simulink model "schemablocpendule1"  (R2021b)
settings: Solver=VariableStepAuto  StartTime=0.0  StopTime=10.0  RelTol=1e-3
undefined symbols (not defined in the file): a, DiscIntNeverNeededParam, Ki, Ku, Ti
libraries: simulink x5, slctrlblks x1
settings Model: Creator=spaet  LastModifiedBy=eloua

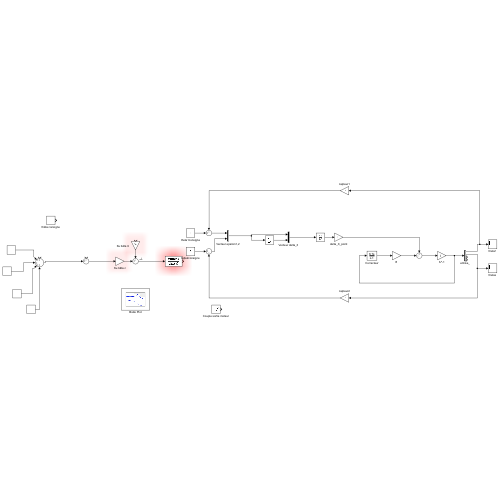
[thumbnail: Simulink's stored preview of the top-level diagram]
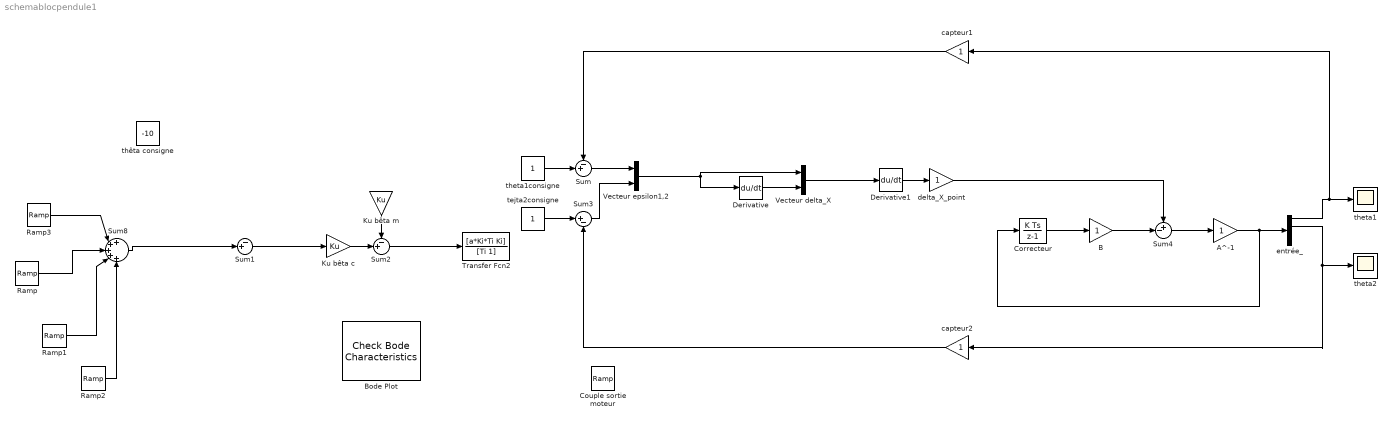
== system schemablocpendule1 ==
  A^-1 : Gain
  B : Gain
  Bode Plot : slctrlblks/Model Verification/Check Bode  Characteristics  InstantiateOnLoad=on  SaveOperatingPoints=off  LinearizationIOs={'/Sum2', 1, 'in', 'on', '';'/TMD sur la caméra', 1, 'out', 'on', ''}  LinearizeAt=SnapshotTimes  SnapshotTimes=[0]  TriggerType=rising  SampleTime=auto  RateConversionMethod=zoh  PreWarpFreq=10  UseExactDelayModel=off  UseFullBlockNameLabels=off  UseBusSignalLabels=off  enabled=on  stopWhenAssertionFail=off  export=off  ViewDlgPos=[137 244 510 390]  OpenViewOnLoad=off  LaunchViewOnOpen=off  FrequencyUnits=rad/s  MagnitudeUnits=dB  PhaseUnits=deg  TimeUnits=seconds  EnableUpperBound=off  UpperBoundFrequencies=[]  UpperBoundMagnitudes=[]  EnableLowerBound=off  LowerBoundFrequencies=[]  LowerBoundMagnitudes=[]
  Correcteur : DiscreteIntegrator  SampleTime=-1  ICPrevOutput=DiscIntNeverNeededParam  ICPrevScaledInput=DiscIntNeverNeededParam
  Couple sortie moteur : simulink/Sources/Ramp  slope=1  start=0  InitialOutput=0
  Derivative : Derivative
  Derivative1 : Derivative
  Ku bêta c : Gain  Gain=Ku
  Ku bêta m : Gain  Gain=Ku
  Ramp : simulink/Sources/Ramp  slope=1  start=0  InitialOutput=0
  Ramp1 : simulink/Sources/Ramp  slope=-1  start=10  InitialOutput=0
  Ramp2 : simulink/Sources/Ramp  slope=-1  start=20  InitialOutput=0
  Ramp3 : simulink/Sources/Ramp  slope=1  start=25  InitialOutput=0
  Sum : Sum  Inputs=-+|
  Sum1 : Sum  Inputs=-+|
  Sum2 : Sum  Inputs=-+|
  Sum3 : Sum  Inputs=|+-
  Sum4 : Sum  Inputs=+-|
  Sum8 : Sum  Inputs=+++++
  Transfer Fcn2 : TransferFcn  Numerator=[a*Ki*Ti Ki]  Denominator=[Ti 1]
  Vecteur delta_X : Mux  Inputs=2
  Vecteur epsilon1,2 : Mux  Inputs=2
  capteur1 : Gain
  capteur2 : Gain
  delta_X_point : Gain
  entrée_ : Demux
  tejta2consigne : Constant
  theta1 : Scope
  theta1consigne : Constant
  theta2 : Scope
  thêta consigne : Constant  Value=-10
  wires:
  Sum1/1 -> Ku bêta c/1
  Ramp3/1 -> Sum8/2
  Sum2/1 -> Transfer Fcn2/1
  Ramp2/1 -> Sum8/5
  Sum8/1 -> Sum1/2
  Ku bêta c/1 -> Sum2/2
  Ramp/1 -> Sum8/3
  Ramp1/1 -> Sum8/4
  Ku bêta m/1 -> Sum2/1
  Vecteur epsilon1,2/1 -> Vecteur delta_X/1, Derivative/1
  Derivative/1 -> Vecteur delta_X/2
  Vecteur delta_X/1 -> Derivative1/1
  Derivative1/1 -> delta_X_point/1
  entrée_/1 -> capteur1/1, theta1/1
  entrée_/2 -> theta2/1, capteur2/1
  theta1consigne/1 -> Sum/2
  Sum/1 -> Vecteur epsilon1,2/1
  tejta2consigne/1 -> Sum3/1
  capteur1/1 -> Sum/1
  capteur2/1 -> Sum3/2
  Sum3/1 -> Vecteur epsilon1,2/2
  A^-1/1 -> Correcteur/1, entrée_/1
  delta_X_point/1 -> Sum4/1
  Sum4/1 -> A^-1/1
  B/1 -> Sum4/2
  Correcteur/1 -> B/1
